simulink model "hw5_p3_open_loop_model_SKELETON"  (R2024a)
settings: Solver=FixedStepAuto  StartTime=0.0  StopTime=tFinal_s  FixedStep=deltaT_s  RelTol=1e-3
values from neighbouring files (symbols this model uses):
  deltaT_s = 0.01    [hw5_p3_SKELETON.m]
  K = 49    [hw5_p3_SKELETON.m]
  noisePower = .00001    (= 1e-05)    [hw5_p3_SKELETON.m]
  Tambient_C = 24.1875    [hw5_p3_SKELETON.m]
  Tdelay_s = 1.2    [hw5_p3_SKELETON.m]
  wn = 0.03    [hw5_p3_SKELETON.m]
  zeta = 1.5    [hw5_p3_SKELETON.m]
libraries: simulink x1
settings Model: PacingRate=3  Creator=chris  LastModifiedBy=chris

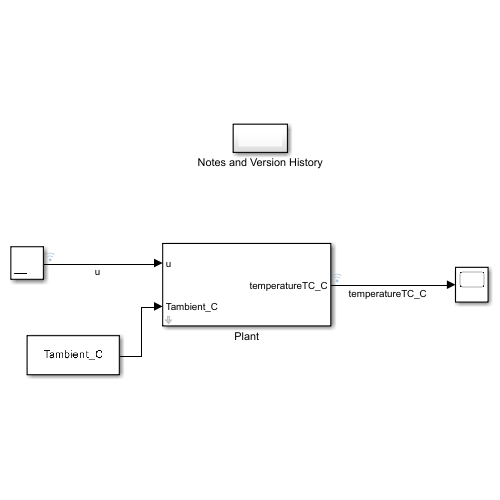
[thumbnail: Simulink's stored preview of the top-level diagram]
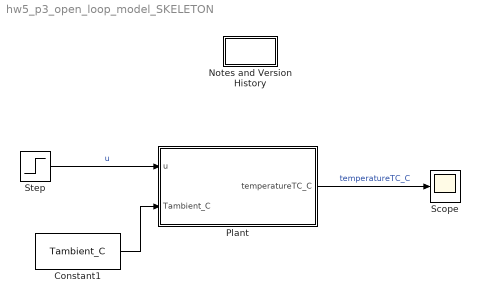
== system hw5_p3_open_loop_model_SKELETON ==
  Constant1 : Constant  Value=Tambient_C
  Notes and Version History : Subsystem
  Plant : Subsystem  mask{wn=wn, zeta=zeta, K=K, Tdelay_s=Tdelay_s, noisePower=noisePower, Tsample_s=deltaT_s}
      mask prompts: Tdelay_s "Delay time (sec)"; noisePower "Noise power"; Tsample_s "Sample Time"
      mask help:
      | Simple first order temperature model
      |
      | Input
      | u = duty cycle (0 = off, 1 = full on)
      |
      | Output
      | temperatureTC_C = temperature (C)
  Scope : Scope
  Step : Step  Time=60  SampleTime=0
  wires:
  Plant/1(temperatureTC_C) -> Scope/1  "temperatureTC_C"
  Constant1/1 -> Plant/2(Tambient_C)
  Step/1 -> Plant/1(u)  "u"

== system hw5_p3_open_loop_model_SKELETON/Notes and Version History ==
  note: Skeleton model for thermal system used for homework.
      |
      | Christopher Lum
      | lum@uw.edu
      |
      | Version History
      | 02/05/25: Created

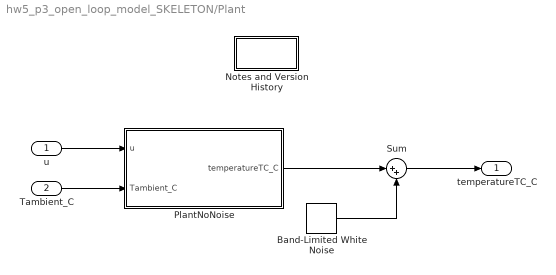
== system hw5_p3_open_loop_model_SKELETON/Plant ==
  u : Inport
  Tambient_C : Inport  Port=2
  Band-Limited White Noise : simulink/Sources/Band-Limited White Noise  Cov=noisePower  Ts=Tsample_s  seed=[23341]
  Notes and Version History : Subsystem
  PlantNoNoise : Subsystem  mask{wn=wn, zeta=zeta, K=K, Tdelay_s=Tdelay_s}
      mask prompts: Tdelay_s "Delay time (sec)"
      mask help:
      | Simple first order temperature model
      |
      | Input
      | u = duty cycle (0 = off, 1 = full on)
      |
      | Output
      | temperatureTC_C = temperature (C)
  Sum : Sum  Inputs=|++
  temperatureTC_C : Outport
  wires:
  Sum/1 -> temperatureTC_C/1
  Band-Limited White Noise/1 -> Sum/2
  PlantNoNoise/1(temperatureTC_C) -> Sum/1
  Tambient_C/1 -> PlantNoNoise/2(Tambient_C)
  u/1 -> PlantNoNoise/1(u)

== system hw5_p3_open_loop_model_SKELETON/Plant/Notes and Version History ==
  note: Similar to PlantType03 but includes a noise model for the sensor output.
      |
      | Christopher Lum
      | lum@uw.edu
      |
      | Version History
      | 01/26/25: Created

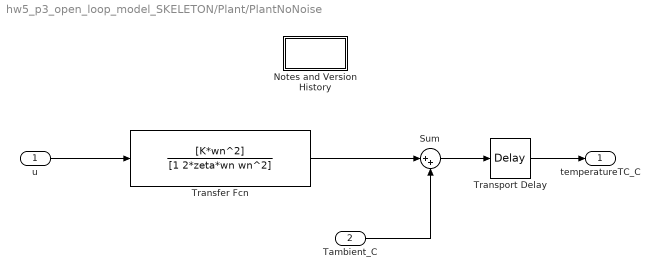
== system hw5_p3_open_loop_model_SKELETON/Plant/PlantNoNoise ==
  u : Inport
  Tambient_C : Inport  Port=2
  Notes and Version History : Subsystem
  Sum : Sum  Inputs=|++
  Transfer Fcn : TransferFcn  Numerator=[K*wn^2]  Denominator=[1 2*zeta*wn wn^2]
  Transport Delay : TransportDelay  DelayTime=Tdelay_s
  temperatureTC_C : Outport
  wires:
  Transport Delay/1 -> temperatureTC_C/1
  Transfer Fcn/1 -> Sum/1
  Sum/1 -> Transport Delay/1
  Tambient_C/1 -> Sum/2
  u/1 -> Transfer Fcn/1

== system hw5_p3_open_loop_model_SKELETON/Plant/PlantNoNoise/Notes and Version History ==
  note: Plant used for simulation
      |
      | Christopher Lum
      | lum@uw.edu
      |
      | Version History
      | 01/24/25: Created
